simulink model "pid1"  (Simulink 3.00)
settings: Solver=ode45  SolverMode=SingleTasking  StartTime=0.0  StopTime=20  MaxStep=.010  RelTol=1e-3  AbsTol=1e-3
undefined symbols (not defined in the file or in its folder): at, bt, ct, dt
settings Model: TimeSaveName=t  SaveOutput=off

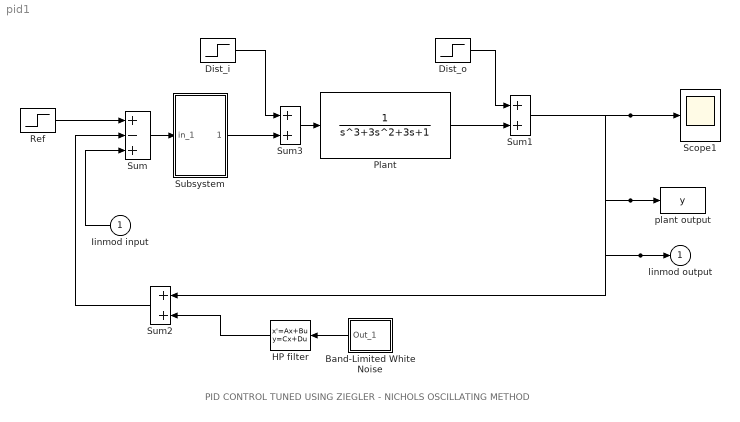
== system pid1 ==
  note: PID CONTROL TUNED USING ZIEGLER - NICHOLS OSCILLATING METHOD
  Iinmod input : Inport  Orientation=left  Port=1  PortWidth=-1  SampleTime=-1  DataType=auto
      settings: SignalType=auto
  Band-Limited White Noise : Subsystem  Orientation=left  mask(Continuous White Noise.){@1=[0], @2=0.1, @3=[23341]}
      mask prompts: @1 "Noise Power:"; @2 "Sample Time:"; @3 "Seed"
      mask help:
      | White noise for continuous (s-domain) systems.
      | Band-limited using zero-order-hold.
      mask init:
      | Cov = @1; Ts = @2; seed = @3; r = rand(1,12); r2 = [r(1),r;r,r(12)]; t =[1:13;1:13];
      mask Help: Implemented using white noise into Zero-Order Hold block. The seed and power can be vectors of the same length to produce a vector of white noise sources. For faster simulation, set sample time to the highest value possible but in accordance with the fastest dynamics of system.
      mask Display: plot(t(:),r2(:))
  Dist_i : Step  Time=10  Before=0  After=1  SampleTime=0
  Dist_o : Step  Time=1  Before=0  After=0  SampleTime=0
  HP filter : StateSpace  Orientation=left  A=at  B=bt  C=ct  D=dt  X0=0  mask(buttap,lp2hp){@1=5, @2=4}
      mask prompts: @1 "Cutoff frequency (rad/sec):"; @2 "Order"
      mask help:
      | Analog Butterworth high pass filter.
      |
      | (Requires Signal Processing Toolbox)
      mask init:
      | [at,bt,ct,dt,w,mag]=filtm('buttap','lp2hp',@1,[],20,@2);
      mask Help: Butterworth high pass filter using MATLAB's butter and lp2hp commands.
      mask Display: plot(w,mag)
  Plant : TransferFcn  Numerator=1  Denominator=[1 3 3 1]
  Ref : Step  Time=0  Before=0  After=1  SampleTime=0
  Scope1 : Scope
      settings: TickLabels=on  TimeRange=20.000000  YMin=-2  YMax=2  SaveToWorkspace=off  SaveName=ScopeData  DataFormat=Matrix
  Subsystem : Subsystem  mask(PID){Kp=4.8, Tr=1.81, Td=0.45, tau_D=0.045}
      mask prompts: Kp "Prop gain:"; Tr "Integral time:"; Td "Derivative time:"; tau_D "Derivative time constant:"
      mask help: PID
      mask Display: disp('PID')
  Sum : Sum  Inputs=+-+  SaturateOnIntegerOverflow=on
  Sum1 : Sum  Inputs=++  SaturateOnIntegerOverflow=on
  Sum2 : Sum  Orientation=left  Inputs=++  SaturateOnIntegerOverflow=on
  Sum3 : Sum  Inputs=++  SaturateOnIntegerOverflow=on
  plant output : ToWorkspace  VariableName=y  SampleTime=0  SaveFormat=Matrix
      settings: Buffer=6000
  linmod output : Outport  Port=1  InitialOutput=0
  wires:
  Plant/1 -> Sum1/2
  Ref/1 -> Sum/1
  Sum1/1 -> Scope1/1, plant output/1, Sum2/1, linmod output/1
  Dist_o/1 -> Sum1/1
  Sum3/1 -> Plant/1
  Dist_i/1 -> Sum3/1
  Subsystem/1(out_1) -> Sum3/2
  Iinmod input/1 -> Sum/3
  Sum/1 -> Subsystem/1(in_1)
  HP filter/1 -> Sum2/2
  Sum2/1 -> Sum/2
  Band-Limited White Noise/1(Out_1) -> HP filter/1

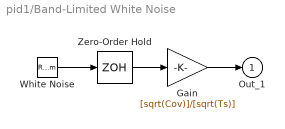
== system pid1/Band-Limited White Noise ==
  Gain : Gain  Gain=[sqrt(Cov)]/[sqrt(Ts)]  SaturateOnIntegerOverflow=on
  White Noise : RandomNumber  Mean=0  Variance=1  Seed=seed  SampleTime=0
  Zero-Order Hold : ZeroOrderHold  SampleTime=Ts
  Out_1 : Outport  Port=1  InitialOutput=0
  wires:
  White Noise/1 -> Zero-Order Hold/1
  Gain/1 -> Out_1/1
  Zero-Order Hold/1 -> Gain/1

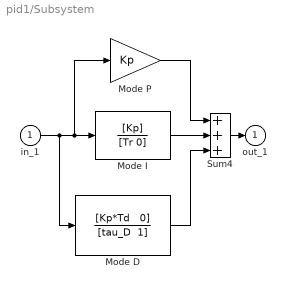
== system pid1/Subsystem ==
  in_1 : Inport  Port=1  PortWidth=-1  SampleTime=-1  DataType=auto
      settings: SignalType=auto
  Mode D : TransferFcn  Numerator="[Kp*Td   0]"  Denominator="[tau_D  1]"
  Mode I : TransferFcn  Numerator=[Kp]  Denominator=[Tr 0]
  Mode P : Gain  Gain=Kp  SaturateOnIntegerOverflow=on
  Sum4 : Sum  Inputs=+++  SaturateOnIntegerOverflow=on
  out_1 : Outport  Port=1  InitialOutput=0
  wires:
  in_1/1 -> Mode D/1, Mode I/1, Mode P/1
  Mode D/1 -> Sum4/3
  Mode P/1 -> Sum4/1
  Mode I/1 -> Sum4/2
  Sum4/1 -> out_1/1
